simulink library "ITKLib"  (R2022b)
settings: Solver=FixedStepDiscrete  StartTime=0.0  StopTime=10.0  FixedStep=0.01  RelTol=1e-3  EnableMultiTasking=on
values from neighbouring files (symbols this model uses):
  Glb_WhlRollgRd_SC = single(0.36)    [init_Global.m]
undefined symbols (not defined in the file or in its folder): docblock, SlDemoSign, SlDemoSign_Positive_SC, TaskTime_100ms_SC, TaskTime_10ms_SC, VehRefSpd_vMaxRefSpd_C
libraries: simulink x51, $bdroot x45, ITKLib_V14 x1
(part 10 of 10)

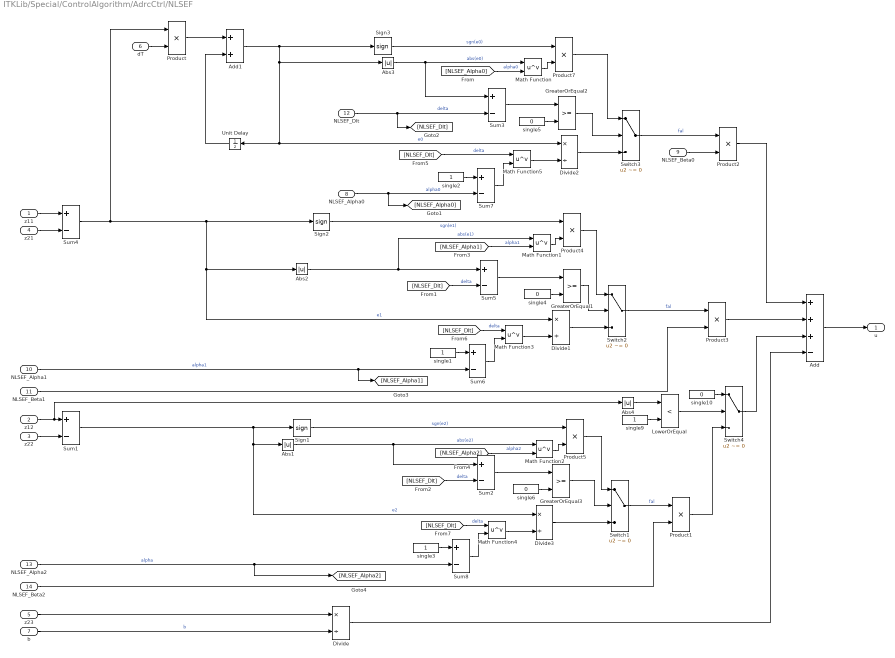
== system ITKLib/Special/ControlAlgorithm/AdrcCtrl/NLSEF ==
  z11 : Inport
  z12 : Inport  Port=2
  z22 : Inport  Port=3
  z21 : Inport  Port=4
  z23 : Inport  Port=5
  dT : Inport  Port=6
  b : Inport  Port=7
  NLSEF_Alpha0 : Inport  Port=8
  NLSEF_Beta0 : Inport  Port=9
  NLSEF_Alpha1 : Inport  Port=10
  NLSEF_Beta1 : Inport  Port=11
  NLSEF_Dlt : Inport  Port=12
  NLSEF_Alpha2 : Inport  Port=13
  NLSEF_Beta2 : Inport  Port=14
  Abs{1..4} (4 alike) : Abs  SaturateOnIntegerOverflow=off
  Add : Sum  Inputs=+++-
  Add1 : Sum
  Divide{,1..3} (4 alike) : Product  Inputs=*/  InputSameDT=on  SaturateOnIntegerOverflow=on
  GreaterOrEqual1 : RelationalOperator  OutDataTypeStr=boolean
  GreaterOrEqual2 : RelationalOperator  OutDataTypeStr=boolean
  GreaterOrEqual3 : RelationalOperator  OutDataTypeStr=boolean
  LowerOrEqual : RelationalOperator  Operator=<  OutDataTypeStr=boolean
  Math Function{,1..5} (6 alike) : Math  Operator=pow
  Product : Product  InputSameDT=on  SaturateOnIntegerOverflow=on
  Product1 : Product  RndMeth=Zero
  Product2 : Product  RndMeth=Zero
  Product3 : Product  RndMeth=Zero
  Product4 : Product
  Product5 : Product
  Product7 : Product
  Sign1 : Signum
  Sign2 : Signum
  Sign3 : Signum
  Sum{1..8} (8 alike) : Sum  Inputs=+-  SaturateOnIntegerOverflow=on
  Switch{1..4} (4 alike) : Switch  Criteria=u2 ~= 0  SaturateOnIntegerOverflow=off  InputSameDT=off
      Switch4 settings: AttributesFormatString=Criteria : %<Criteria>
  Unit Delay : UnitDelay  SampleTime=-1  HasFrameUpgradeWarning=on
  single{1..3,9} (4 alike) : Constant  OutDataTypeStr=single  SampleTime=-1
      settings: AttributesFormatString=%<OutDataTypeStr>
  single{4..6,10} (4 alike) : Constant  Value=0  OutDataTypeStr=single  SampleTime=-1
      settings: AttributesFormatString=%<OutDataTypeStr>
  u : Outport  VectorParamsAs1DForOutWhenUnconnected=off
  wires:
  Switch2/1 -> Product3/1  "fal"
  NLSEF_Alpha1/1 -> [NLSEF_Alpha1], Sum6/2  "alpha1"
  Product4/1 -> Switch2/1
  Abs2/1 -> Math Function1/1, Sum5/1  "abs(e1)"
  Divide1/1 -> Switch2/3
  Sum5/1 -> GreaterOrEqual1/1
  z11/1 -> Sum4/1
  [NLSEF_Dlt] -> Sum5/2  "delta"
  Sum4/1 -> Product/1, Sign2/1, Divide1/1, Abs2/1  "e1"
  Sign2/1 -> Product4/1  "sgn(e1)"
  NLSEF_Beta1/1 -> Product3/2
  z21/1 -> Sum4/2
  z22/1 -> Sum1/2
  NLSEF_Beta2/1 -> Product1/2
  Sign1/1 -> Product5/1  "sgn(e2)"
  Sum1/1 -> Sign1/1, Divide3/1, Abs1/1  "e2"
  [NLSEF_Dlt] -> Sum2/2  "delta"
  Divide3/1 -> Switch1/3
  Abs1/1 -> Math Function2/1, Sum2/1  "abs(e2)"
  NLSEF_Alpha2/1 -> [NLSEF_Alpha2], Sum8/2  "alpha"
  Sum2/1 -> GreaterOrEqual3/1
  Switch1/1 -> Product1/1  "fal"
  z12/1 -> Abs4/1, Sum1/1
  Product1/1 -> Switch4/3
  Product3/1 -> Add/2
  Product2/1 -> Add/1
  z23/1 -> Divide/1
  Divide/1 -> Add/4
  Add/1 -> u/1
  NLSEF_Dlt/1 -> Sum3/2, [NLSEF_Dlt]  "delta"
  Sign3/1 -> Product7/1  "sgn(e0)"
  NLSEF_Beta0/1 -> Product2/2
  Product7/1 -> Switch3/1
  Add1/1 -> Unit Delay/1, Divide2/1, Abs3/1, Sign3/1  "e0"
  Abs3/1 -> Math Function/1, Sum3/1  "abs(e0)"
  Sum3/1 -> GreaterOrEqual2/1
  Divide2/1 -> Switch3/3
  NLSEF_Alpha0/1 -> [NLSEF_Alpha0], Sum7/2  "alpha0"
  Switch3/1 -> Product2/1  "fal"
  [NLSEF_Alpha0] -> Math Function/2  "alpha0"
  [NLSEF_Alpha1] -> Math Function1/2  "alpha1"
  [NLSEF_Alpha2] -> Math Function2/2  "alpha2"
  b/1 -> Divide/2  "b"
  Unit Delay/1 -> Add1/2
  Product/1 -> Add1/1
  dT/1 -> Product/2
  Math Function/1 -> Product7/2
  Math Function1/1 -> Product4/2
  Math Function2/1 -> Product5/2
  Product5/1 -> Switch1/1
  single2/1 -> Sum7/1
  Math Function5/1 -> Divide2/2
  Sum7/1 -> Math Function5/2
  [NLSEF_Dlt] -> Math Function5/1  "delta"
  Sum6/1 -> Math Function3/2
  Math Function3/1 -> Divide1/2
  single1/1 -> Sum6/1
  [NLSEF_Dlt] -> Math Function3/1  "delta"
  [NLSEF_Dlt] -> Math Function4/1  "delta"
  single3/1 -> Sum8/1
  Math Function4/1 -> Divide3/2
  Sum8/1 -> Math Function4/2
  single5/1 -> GreaterOrEqual2/2
  GreaterOrEqual2/1 -> Switch3/2
  single4/1 -> GreaterOrEqual1/2
  GreaterOrEqual1/1 -> Switch2/2
  single6/1 -> GreaterOrEqual3/2
  GreaterOrEqual3/1 -> Switch1/2
  single10/1 -> Switch4/1
  LowerOrEqual/1 -> Switch4/2
  single9/1 -> LowerOrEqual/2
  Abs4/1 -> LowerOrEqual/1
  Switch4/1 -> Add/3

== system ITKLib/Special/ControlAlgorithm/AdrcCtrl/TD ==
  yd : Inport
  r : Inport  Port=2
  h : Inport  Port=3
  Ts : Inport  Port=4
  Abs : Abs  SaturateOnIntegerOverflow=off
  Abs1 : Abs  SaturateOnIntegerOverflow=off
  Add{,1..3} (4 alike) : Sum
  Divide : Product  Inputs=*/
  Divide1 : Product  Inputs=**/
  Divide2 : Product  Inputs=*/
  Gain : Gain  Gain=-1
  Gain1 : Gain  Gain=-1
  GreaterOrEqual1 : RelationalOperator  OutDataTypeStr=boolean
  GreaterOrEqual2 : RelationalOperator  OutDataTypeStr=boolean
  Product{,1..6,8} (8 alike) : Product  RndMeth=Zero
  Product7 : Product  Inputs=3  RndMeth=Zero
  Sign : Signum
  Sign1 : Signum
  Sqrt : $bdroot/BasicOperators/Sqrt
  Sum1 : Sum  Inputs=+-+  SaturateOnIntegerOverflow=on
  Sum2 : Sum  Inputs=+-  SaturateOnIntegerOverflow=on
  Sum3 : Sum  Inputs=+-  SaturateOnIntegerOverflow=on
  Sum4 : Sum  Inputs=+-  SaturateOnIntegerOverflow=on
  Switch : Switch  Criteria=u2 ~= 0  SaturateOnIntegerOverflow=off  InputSameDT=off
  Switch1 : Switch  Criteria=u2 ~= 0  SaturateOnIntegerOverflow=off  InputSameDT=off
  Unit Delay : UnitDelay  SampleTime=-1  HasFrameUpgradeWarning=on
  Unit Delay1 : UnitDelay  SampleTime=-1  HasFrameUpgradeWarning=on
  single : Constant  Value=2  OutDataTypeStr=single  SampleTime=-1
      settings: AttributesFormatString=%<OutDataTypeStr>
  single1 : Constant  Value=8  OutDataTypeStr=single  SampleTime=-1
      settings: AttributesFormatString=%<OutDataTypeStr>
  single2 : Constant  Value=0  OutDataTypeStr=single  SampleTime=-1
      settings: AttributesFormatString=%<OutDataTypeStr>
  single5 : Constant  Value=0  OutDataTypeStr=single  SampleTime=-1
      settings: AttributesFormatString=%<OutDataTypeStr>
  z11 : Outport  VectorParamsAs1DForOutWhenUnconnected=off
  z12 : Outport  Port=2  VectorParamsAs1DForOutWhenUnconnected=off
  wires:
  Product/1 -> Sum4/2, Product8/2, Product8/1, Divide1/3, Sum3/2, Product1/1  "d"
  r/1 -> [r], Product/1  "r"
  Switch1/1 -> Product4/1  "fhan"
  Add/1 -> Unit Delay/1  "y2(k+1)"
  h/1 -> Product/2, [h], Product3/2  "h"
  Abs/1 -> Product7/2, [y0abs]  "abs(y0)"
  Sum2/1 -> GreaterOrEqual2/1
  Sum3/1 -> GreaterOrEqual1/1
  Divide1/1 -> Gain1/1
  Product2/1 -> Gain/1
  Gain/1 -> Switch1/1
  yd/1 -> Sum1/2
  Sign1/1 -> Product2/1  "sgn(a)"
  Divide/1 -> Switch/3
  Sum1/1 -> [y0], Abs/1  "y0"
  Add2/1 -> Divide1/2, Abs1/1, Sign1/1  "a"
  Abs1/1 -> Sum3/1  "abs(a)"
  Sign/1 -> Product6/2  "sgn(y0)"
  Product1/1 -> Sum2/2  "d0"
  Sqrt/1 -> Sum4/1  "a0"
  Gain1/1 -> Switch1/3
  Product4/1 -> Add/1
  Unit Delay/1 -> Add/2, z12/1, [y2k]  "y2(k)"
  [y2k] -> Product5/1
  Product5/1 -> Add1/1
  Add1/1 -> Unit Delay1/1  "y1(k+1)"
  Unit Delay1/1 -> Add1/2, Sum1/1, z11/1  "y1(k)"
  [y2k] -> Product3/1
  Product3/1 -> Sum1/3
  Divide2/1 -> Switch/1
  Switch/1 -> Add2/2
  [y2k] -> Add2/1
  [y0abs] -> Sum2/1
  [y0] -> Sign/1
  [y0] -> Divide/1
  [r] -> Product2/2  "r"
  [r] -> Divide1/1  "r"
  [h] -> Divide/2, Product1/2  "h"
  Ts/1 -> [Ts], Product4/2
  [Ts] -> Product5/2
  Sum4/1 -> Product6/1
  Product6/1 -> Divide2/1
  single/1 -> Divide2/2
  single1/1 -> Product7/1
  Product7/1 -> Add3/1
  Product8/1 -> Add3/2
  Add3/1 -> Sqrt/1
  [r] -> Product7/3  "r"
  single5/1 -> GreaterOrEqual2/2
  GreaterOrEqual2/1 -> Switch/2
  single2/1 -> GreaterOrEqual1/2
  GreaterOrEqual1/1 -> Switch1/2

== system ITKLib/Special/ControlAlgorithm/RCCritCurr/Safe_Divide ==
  In : Inport
  In1 : Inport  Port=2
  eps : Inport  Port=3
  AND : Logic  OutDataTypeStr=boolean
  Abs : Abs  SaturateOnIntegerOverflow=off  OutDataTypeStr=Inherit: Inherit via internal rule
  Divide : Product  Inputs=*/  InputSameDT=on  SaturateOnIntegerOverflow=on
  GreaterOrEqual : RelationalOperator  OutDataTypeStr=boolean
  GreaterOrEqual1 : RelationalOperator  OutDataTypeStr=boolean
  LowerOrEqual : RelationalOperator  Operator=<=  OutDataTypeStr=boolean
  Opposite : Subsystem  RTWFcnName=Minus  RTWFileName=MCC_Mdl_Lib  mask(Opposite){}
      mask help:
      | output = - input;
      | Simulink Custom Model Library, created by MCC.
      settings: RTWFcnNameOpts=User specified  RTWFileNameOpts=User specified
      mask Display:
      | color('blue')
      | fprintf('-ln  ')
      | color('green');
      | % text(1,0,'SEN','horizontalAlignment','right','verticalAlignment','bottom');
  Opposite1 : Subsystem  RTWFcnName=Minus  RTWFileName=MCC_Mdl_Lib  mask(Opposite){}
      mask help:
      | output = - input;
      | Simulink Custom Model Library, created by MCC.
      settings: RTWFcnNameOpts=User specified  RTWFileNameOpts=User specified
      mask Display:
      | color('blue')
      | fprintf('-ln  ')
      | color('green');
      | % text(1,0,'SEN','horizontalAlignment','right','verticalAlignment','bottom');
  Switch : Switch  Criteria=u2 ~= 0  SaturateOnIntegerOverflow=off  InputSameDT=off
      settings: AttributesFormatString=Criteria : %<Criteria>
  Switch1 : Switch  Criteria=u2 ~= 0  SaturateOnIntegerOverflow=off  InputSameDT=off
      settings: AttributesFormatString=Criteria : %<Criteria>
  single : Constant  Value=0  OutDataTypeStr=single
      settings: AttributesFormatString=%<OutDataTypeStr>
  Out : Outport
  wires:
  Divide/1 -> Out/1
  In/1 -> Divide/1
  Switch/1 -> Divide/2
  AND/1 -> Switch/2
  In1/1 -> GreaterOrEqual/1, Switch/3, LowerOrEqual/1, GreaterOrEqual1/1
  single/1 -> GreaterOrEqual1/2
  eps/1 -> Abs/1
  Abs/1 -> [epsAbs], LowerOrEqual/2
  LowerOrEqual/1 -> AND/1
  GreaterOrEqual/1 -> AND/2
  Opposite/1(" Out ") -> GreaterOrEqual/2
  [epsAbs] -> Opposite/1(In)
  GreaterOrEqual1/1 -> Switch1/2
  [epsAbs] -> Opposite1/1(In)
  Opposite1/1(" Out ") -> Switch1/3
  [epsAbs] -> Switch1/1
  Switch1/1 -> Switch/1

== system ITKLib/Special/ControlAlgorithm/RCCritCurr/Safe_Divide/Opposite ==
  In : Inport
  Product2 : Product  InputSameDT=on  SaturateOnIntegerOverflow=on
  single : Constant  Value=-1  OutDataTypeStr=single
      settings: AttributesFormatString=%<OutDataTypeStr>
  " Out " : Outport
  wires:
  single/1 -> Product2/2
  Product2/1 -> " Out "/1
  In/1 -> Product2/1

== system ITKLib/Special/ControlAlgorithm/RCCritCurr/Safe_Divide/Opposite1 ==
  In : Inport
  Product2 : Product  InputSameDT=on  SaturateOnIntegerOverflow=on
  single : Constant  Value=-1  OutDataTypeStr=single
      settings: AttributesFormatString=%<OutDataTypeStr>
  " Out " : Outport
  wires:
  single/1 -> Product2/2
  Product2/1 -> " Out "/1
  In/1 -> Product2/1

== stateflow chart ITKLib/BasicOperators/Chart ==
  settings: updateMethod=DISCRETE

== matlab function ITKLib/Diagnosis/Crc8Gen ==
  data: MsgData input; CRCVal output; ChkLen input; Poly input; InitVal input; XORVal input
%% CRC8校验算法：生成CRC8 Checksum的Value数值
% Input signals：
%               MsgData:包含8个byte的完整的一个ID的报文数据包
%               ChkLen:进行校验的ID数据长度对应的数值，通常为固定值7个byte对应01111111对应的uint8为127
%               Poly:多项式Polynomial值，此处可以设置为16进制对应的十进制uint8数值
%               InitVal:初始值，此处可以设置为16进制对应的十进制uint8数值
%               XORVal:结果异或值XOROUT，此处可以设置为16进制对应的十进制uint8数值

%% 主函数
function CRCVal = Crc8Gen(MsgData,ChkLen,Poly,InitVal,XORVal)
crc = InitVal;
for i = 1:length(MsgData)
    if bitget(ChkLen,i) == 1
        crc = bitxor(crc,MsgData(i));
        for j = 0:7
            if bitand(crc,0x80) ~= 0
                crc = bitxor(bitshift(crc,1),Poly);
            else
                crc = bitshift(crc,1); 
            end
        end
    end
end
CRCVal = bitxor(crc,XORVal);
end

== matlab function ITKLib/BitOperation/GetBitU16/MATLAB Function ==
  data: u input; y output; mode input; N input
function y = fcn(u, mode, N)
%#codegen

switch mode
    case 1 % 逻辑左移 Shift Left Logical
        y = bitsll(cast_to_fi(u), N);
    case 2  % 逻辑右移 Shift Right Logical
        y = bitsrl(cast_to_fi(u), N);
%     case 3 % 算数右移 Shift Right Arithmetic
%         y = bitsra(cast_to_fi(u), N);
    otherwise
        y = cast_to_fi(u);
end

== matlab function ITKLib/BitOperation/GetBitU16/MATLAB Function1 ==
  data: u input; y output; mode input; N input
function y = fcn(u, mode, N)
%#codegen

switch mode
    case 1 % 逻辑左移 Shift Left Logical
        y = bitsll(cast_to_fi(u), N);
    case 2  % 逻辑右移 Shift Right Logical
        y = bitsrl(cast_to_fi(u), N);
%     case 3 % 算数右移 Shift Right Arithmetic
%         y = bitsra(cast_to_fi(u), N);
    otherwise
        y = cast_to_fi(u);
end

== matlab function ITKLib/BitOperation/GetBitU8/MATLAB Function ==
  data: u input; y output; mode input; N input
function y = fcn(u, mode, N)
%#codegen

switch mode
    case 1 % 逻辑左移 Shift Left Logical，尽量选择逻辑左移或右移
        y = bitsll(cast_to_fi(u), N);
    case 2  % 逻辑右移 Shift Right Logical
        y = bitsrl(cast_to_fi(u), N);
%     case 3 % 算数右移 Shift Right Arithmetic
%         y = bitsra(cast_to_fi(u), N);
    otherwise
        y = cast_to_fi(u);
end

== matlab function ITKLib/BitOperation/GetBitU8/MATLAB Function1 ==
  data: u input; y output; mode input; N input
function y = fcn(u, mode, N)
%#codegen

switch mode
    case 1 % 逻辑左移 Shift Left Logical
        y = bitsll(cast_to_fi(u), N);
    case 2  % 逻辑右移 Shift Right Logical
        y = bitsrl(cast_to_fi(u), N);
%     case 3 % 算数右移 Shift Right Arithmetic
%         y = bitsra(cast_to_fi(u), N);
    otherwise
        y = cast_to_fi(u);
end

== matlab function ITKLib/BitOperation/GetBitU32/MATLAB Function ==
  data: u input; y output; mode input; N input
function y = fcn(u, mode, N)
%#codegen

switch mode
    case 1 % 逻辑左移 Shift Left Logical
        y = bitsll(cast_to_fi(u), N);
    case 2  % 逻辑右移 Shift Right Logical
        y = bitsrl(cast_to_fi(u), N);
%     case 3 % 算数右移 Shift Right Arithmetic
%         y = bitsra(cast_to_fi(u), N);
    otherwise
        y = cast_to_fi(u);
end

== matlab function ITKLib/BitOperation/GetBitU32/MATLAB Function1 ==
  data: u input; y output; mode input; N input
function y = fcn(u, mode, N)
%#codegen

switch mode
    case 1 % 逻辑左移 Shift Left Logical
        y = bitsll(cast_to_fi(u), N);
    case 2  % 逻辑右移 Shift Right Logical
        y = bitsrl(cast_to_fi(u), N);
%     case 3 % 算数右移 Shift Right Arithmetic
%         y = bitsra(cast_to_fi(u), N);
    otherwise
        y = cast_to_fi(u);
end

== stateflow chart ITKLib/Filter/MovgMinMaxAvrg ==
  (default) -> (junction 40) : {
      | /* Buffer new running average result */
      | InBufAry[idx] = In;
      | /* Increment persistent buffer pointer */
      | idx++;
      | /* Initialise FOR loop */
      | idx_loop = uint16(0);
      | Min = single(999999999999999999);
      | Max = single(-999999999999999999);
      | Avrg = single(0);
      | Sum = single(0);
      | }
  (junction 40) -> (junction 54) [order 1] : [idx_loop < DataNr]
  (junction 54) -> (junction 53) [order 1] : [InBufAry[idx_loop] > Max]
  (junction 102) -> (junction 40) : {idx_loop++;}
  (junction 40) -> (junction 7) [order 2] : {
      | /* Average the totals for input */
      | Avrg = Sum / DataNr;
      | }
  (junction 54) -> (junction 103) [order 2]
  (junction 53) -> (junction 52) : {
      | Max = InBufAry[idx_loop];
      | }
  (junction 103) -> (junction 105) [order 1] : [InBufAry[idx_loop] < Min]
  (junction 103) -> (junction 55) [order 2]
  (junction 105) -> (junction 107) : {
      | Min = InBufAry[idx_loop];
      | }
  (junction 107) -> (junction 55)
  (junction 52) -> (junction 107)
  (junction 55) -> (junction 102) : {
      | Sum = Sum+InBufAry[idx_loop];
      | }
  (junction 7) -> (junction 10) [order 1] : /* Ring buffer pointer has reached end of ring */
      | [idx == DataNr]
  (junction 7) -> (junction 9) [order 2]
  (junction 10) -> (junction 11) : /* Reset pointer to start of buffer */
      | {idx = uint16(0);}
  (junction 11) -> (junction 9)
  data: In input single; InBufAry local single size=[1 DataNr]; idx local uint16 size=1 =0; DataNr input uint16; idx_loop local uint16 size=1 =0; Sum local single; Min output single; Max output single; Avrg output single; data local single

== stateflow chart ITKLib/TimeCounter/trig_TaskTime_A ==
  settings: updateMethod=DISCRETE
  (default) -> (junction 52) : {cnt = cnt + 1;}
  (junction 52) -> (junction 54) [order 1] : [cnt %% 2 == 0]
  (junction 52) -> (junction 58) [order 2]
  (junction 54) -> (junction 56) : {
      |   trig_TaskTime_20ms;
      | }
  (junction 56) -> (junction 58)
  (junction 58) -> (junction 83)
  (junction 83) -> (junction 81) [order 1] : [cnt %% 5 == 0]
  (junction 83) -> (junction 87) [order 2]
  (junction 81) -> (junction 82) : {
      |   trig_TaskTime_50ms;
      | }
  (junction 82) -> (junction 87)
  (junction 87) -> (junction 96)
  (junction 96) -> (junction 90) [order 1] : [cnt %% 10 == 0]
  (junction 96) -> (junction 95) [order 2]
  (junction 90) -> (junction 93) : {
      |   trig_TaskTime_100ms;
      | }
  (junction 93) -> (junction 95)
  (junction 95) -> (junction 111)
  (junction 111) -> (junction 114) [order 1] : [cnt %% 20 == 0]
  (junction 111) -> (junction 110) [order 2]
  (junction 114) -> (junction 108) : {
      |   trig_TaskTime_200ms;
      | }
  (junction 108) -> (junction 110)
  (junction 110) -> (junction 118)
  (junction 118) -> (junction 120) [order 1] : [cnt %% 50 == 0]
  (junction 118) -> (junction 117) [order 2]
  (junction 120) -> (junction 124) : {
      |   trig_TaskTime_500ms;
      | }
  (junction 124) -> (junction 117)
  (junction 117) -> (junction 128)
  (junction 128) -> (junction 132) [order 1] : [cnt %% 100 == 0]
  (junction 128) -> (junction 131) [order 2]
  (junction 132) -> (junction 126) : {
      |   trig_TaskTime_1000ms;
      |   cnt = 0;
      | }
  (junction 126) -> (junction 131)
  (junction 131) -> (junction 20)
  data: cnt local uint16
  events: trig_TaskTime_20ms output FUNCTION_CALL_EVENT; trig_TaskTime_50ms output FUNCTION_CALL_EVENT; trig_TaskTime_100ms output FUNCTION_CALL_EVENT; trig_TaskTime_200ms output FUNCTION_CALL_EVENT; trig_TaskTime_500ms output FUNCTION_CALL_EVENT; trig_TaskTime_1000ms output FUNCTION_CALL_EVENT

== stateflow chart ITKLib/TimeCounter/trig_TaskTime_B ==
  settings: updateMethod=DISCRETE
  (default) -> (junction 52) : {cnt = cnt + 1;}
  (junction 52) -> (junction 54) [order 1] : [cnt %% 3 == 0]
  (junction 52) -> (junction 58) [order 2]
  (junction 54) -> (junction 56) : {
      |   trig_TaskTime_30ms;
      | }
  (junction 56) -> (junction 58)
  (junction 58) -> (junction 83)
  (junction 83) -> (junction 81) [order 1] : [cnt %% 15 == 0]
  (junction 83) -> (junction 87) [order 2]
  (junction 81) -> (junction 82) : {
      |   trig_TaskTime_150ms;
      | }
  (junction 82) -> (junction 87)
  (junction 87) -> (junction 96)
  (junction 96) -> (junction 90) [order 1] : [cnt %% 30 == 0]
  (junction 96) -> (junction 95) [order 2]
  (junction 90) -> (junction 93) : {
      |   trig_TaskTime_300ms;
      |   cnt = 0;
      | }
  (junction 93) -> (junction 95)
  (junction 95) -> (junction 20)
  data: cnt local uint16
  events: trig_TaskTime_30ms output FUNCTION_CALL_EVENT; trig_TaskTime_150ms output FUNCTION_CALL_EVENT; trig_TaskTime_300ms output FUNCTION_CALL_EVENT

== stateflow chart ITKLib/Diagnosis/FltCollctn/FltStAry ==
  settings: updateMethod=DISCRETE
  (default) -> (junction 233)
  (junction 233) -> (junction 257) : {BatProt_stFltAry[FltNr-1] = (BatProt_stFltAry[FltNr-1] & 0xFD);}
  (junction 257) -> (junction 265)
  (junction 265) -> (junction 244) : {BatProt_stFltAry[FltNr-1] = (BatProt_stFltAry[FltNr-1] & 0xF7);}
  (junction 244) -> (junction 250)
  (junction 250) -> (junction 266) [order 1] : [FltFlg==1]{BatProt_stFltAry[FltNr-1] = (BatProt_stFltAry[FltNr-1] | 0x10);}
  (junction 250) -> (junction 252) [order 2] : {BatProt_stFltAry[FltNr-1] = (BatProt_stFltAry[FltNr-1] & 0xEF);}
  (junction 266) -> (junction 246)
  (junction 246) -> (junction 252)
  (junction 252) -> (junction 239)
  (junction 239) -> (junction 258) : {BatProt_stFltAry[FltNr-1] = (BatProt_stFltAry[FltNr-1] & 0xFB);}
  data: FltNr input uint8; BatProt_stFltAry data_store_memory size=4; FltFlg input boolean

== stateflow chart ITKLib/Diagnosis/FltCollctn/FltStCodAry ==
  settings: updateMethod=DISCRETE
  (default) -> (junction 13)
  (junction 13) -> (junction 15) [order 1] : [FltFlg]
  (junction 15) -> (junction 19) [order 1] : [BitPos==0]{BatProt_stFltCodAry[AryIdx]=(BatProt_stFltCodAry[AryIdx] | 0x1);}
  (junction 13) -> (junction 136) [order 2]
  (junction 15) -> (junction 22) [order 2]
  (junction 19) -> (junction 21)
  (junction 22) -> (junction 21) [order 1] : [BitPos==1]{BatProt_stFltCodAry[AryIdx]=(BatProt_stFltCodAry[AryIdx] | 0x2);}
  (junction 22) -> (junction 30) [order 2]
  (junction 21) -> (junction 32)
  (junction 136) -> (junction 166) [order 1] : [BitPos==0]{BatProt_stFltCodAry[AryIdx]=(BatProt_stFltCodAry[AryIdx] & 0xFFFE);}
  (junction 30) -> (junction 32) [order 1] : [BitPos==2]{BatProt_stFltCodAry[AryIdx]=(BatProt_stFltCodAry[AryIdx] | 0x4);}
  (junction 136) -> (junction 177) [order 2]
  (junction 166) -> (junction 169)
  (junction 30) -> (junction 39) [order 2]
  (junction 32) -> (junction 36)
  (junction 39) -> (junction 36) [order 1] : [BitPos==3]{BatProt_stFltCodAry[AryIdx]=(BatProt_stFltCodAry[AryIdx] | 0x8);}
  (junction 177) -> (junction 169) [order 1] : [BitPos==1]{BatProt_stFltCodAry[AryIdx]=(BatProt_stFltCodAry[AryIdx] & 0xFFFD);}
  (junction 39) -> (junction 42) [order 2]
  (junction 36) -> (junction 50)
  (junction 177) -> (junction 179) [order 2]
  (junction 169) -> (junction 138)
  (junction 179) -> (junction 138) [order 1] : [BitPos==2]{BatProt_stFltCodAry[AryIdx]=(BatProt_stFltCodAry[AryIdx] & 0xFFFB);}
  (junction 42) -> (junction 50) [order 1] : [BitPos==4]{BatProt_stFltCodAry[AryIdx]=(BatProt_stFltCodAry[AryIdx] | 0x10);}
  (junction 179) -> (junction 122) [order 2]
  (junction 138) -> (junction 163)
  (junction 42) -> (junction 44) [order 2]
  (junction 50) -> (junction 46)
  (junction 122) -> (junction 163) [order 1] : [BitPos==3]{BatProt_stFltCodAry[AryIdx]=(BatProt_stFltCodAry[AryIdx] & 0xFFF7);}
  (junction 44) -> (junction 46) [order 1] : [BitPos==5]{BatProt_stFltCodAry[AryIdx]=(BatProt_stFltCodAry[AryIdx] | 0x20);}
  (junction 122) -> (junction 130) [order 2]
  (junction 163) -> (junction 109)
  (junction 44) -> (junction 45) [order 2]
  (junction 46) -> (junction 49)
  (junction 45) -> (junction 49) [order 1] : [BitPos==6]{BatProt_stFltCodAry[AryIdx]=(BatProt_stFltCodAry[AryIdx] | 0x40);}
  (junction 130) -> (junction 109) [order 1] : [BitPos==4]{BatProt_stFltCodAry[AryIdx]=(BatProt_stFltCodAry[AryIdx] & 0xFFEF);}
  (junction 45) -> (junction 64) [order 2]
  (junction 49) -> (junction 81)
  (junction 130) -> (junction 111) [order 2]
  (junction 109) -> (junction 175)
  (junction 64) -> (junction 81) [order 1] : [BitPos==7]{BatProt_stFltCodAry[AryIdx]=(BatProt_stFltCodAry[AryIdx] | 0x80);}
  (junction 64) -> (junction 67) [order 2]
  (junction 81) -> (junction 75)
  (junction 111) -> (junction 175) [order 1] : [BitPos==5]{BatProt_stFltCodAry[AryIdx]=(BatProt_stFltCodAry[AryIdx] & 0xFFDF);}
  (junction 111) -> (junction 121) [order 2]
  (junction 175) -> (junction 105)
  (junction 67) -> (junction 75) [order 1] : [BitPos==8]{BatProt_stFltCodAry[AryIdx]=(BatProt_stFltCodAry[AryIdx] | 0x100);}
  (junction 67) -> (junction 69) [order 2]
  (junction 75) -> (junction 79)
  (junction 121) -> (junction 105) [order 1] : [BitPos==6]{BatProt_stFltCodAry[AryIdx]=(BatProt_stFltCodAry[AryIdx] & 0xFFBF);}
  (junction 121) -> (junction 104) [order 2]
  (junction 105) -> (junction 143)
  (junction 69) -> (junction 79) [order 1] : [BitPos==9]{BatProt_stFltCodAry[AryIdx]=(BatProt_stFltCodAry[AryIdx] | 0x200);}
  (junction 104) -> (junction 143) [order 1] : [BitPos==7]{BatProt_stFltCodAry[AryIdx]=(BatProt_stFltCodAry[AryIdx] & 0xFF7F);}
  (junction 69) -> (junction 71) [order 2]
  (junction 79) -> (junction 57)
  (junction 104) -> (junction 171) [order 2]
  (junction 143) -> (junction 110)
  (junction 71) -> (junction 57) [order 1] : [BitPos==10]{BatProt_stFltCodAry[AryIdx]=(BatProt_stFltCodAry[AryIdx] | 0x400);}
  (junction 171) -> (junction 110) [order 1] : [BitPos==8]{BatProt_stFltCodAry[AryIdx]=(BatProt_stFltCodAry[AryIdx] & 0xFEFF);}
  (junction 71) -> (junction 59) [order 2]
  (junction 57) -> (junction 63)
  (junction 171) -> (junction 149) [order 2]
  (junction 110) -> (junction 145)
  (junction 59) -> (junction 63) [order 1] : [BitPos==11]{BatProt_stFltCodAry[AryIdx]=(BatProt_stFltCodAry[AryIdx] | 0x800);}
  (junction 149) -> (junction 145) [order 1] : [BitPos==9]{BatProt_stFltCodAry[AryIdx]=(BatProt_stFltCodAry[AryIdx] & 0xFDFF);}
  (junction 59) -> (junction 68) [order 2]
  (junction 63) -> (junction 55)
  (junction 149) -> (junction 176) [order 2]
  (junction 145) -> (junction 131)
  (junction 68) -> (junction 55) [order 1] : [BitPos==12]{BatProt_stFltCodAry[AryIdx]=(BatProt_stFltCodAry[AryIdx] | 0x1000);}
  (junction 176) -> (junction 131) [order 1] : [BitPos==10]{BatProt_stFltCodAry[AryIdx]=(BatProt_stFltCodAry[AryIdx] & 0xFBFF);}
  (junction 68) -> (junction 98) [order 2]
  (junction 55) -> (junction 95)
  (junction 176) -> (junction 142) [order 2]
  (junction 131) -> (junction 106)
  (junction 98) -> (junction 95) [order 1] : [BitPos==13]{BatProt_stFltCodAry[AryIdx]=(BatProt_stFltCodAry[AryIdx] | 0x2000);}
  (junction 142) -> (junction 106) [order 1] : [BitPos==11]{BatProt_stFltCodAry[AryIdx]=(BatProt_stFltCodAry[AryIdx] & 0xF7FF);}
  (junction 98) -> (junction 90) [order 2]
  (junction 95) -> (junction 89)
  (junction 142) -> (junction 103) [order 2]
  (junction 106) -> (junction 146)
  (junction 90) -> (junction 89) [order 1] : [BitPos==14]{BatProt_stFltCodAry[AryIdx]=(BatProt_stFltCodAry[AryIdx] | 0x4000);}
  (junction 103) -> (junction 146) [order 1] : [BitPos==12]{BatProt_stFltCodAry[AryIdx]=(BatProt_stFltCodAry[AryIdx] & 0xEFFF);}
  (junction 90) -> (junction 91) [order 2]
  (junction 89) -> (junction 97)
  (junction 103) -> (junction 118) [order 2]
  (junction 146) -> (junction 178)
  (junction 91) -> (junction 97) [order 1] : [BitPos==15]{BatProt_stFltCodAry[AryIdx]=(BatProt_stFltCodAry[AryIdx] | 0x8000);}
  (junction 118) -> (junction 178) [order 1] : [BitPos==13]{BatProt_stFltCodAry[AryIdx]=(BatProt_stFltCodAry[AryIdx] & 0xDFFF);}
  (junction 91) -> (junction 189) [order 2]
  (junction 97) -> (junction 186)
  (junction 118) -> (junction 173) [order 2]
  (junction 178) -> (junction 134)
  (junction 173) -> (junction 134) [order 1] : [BitPos==14]{BatProt_stFltCodAry[AryIdx]=(BatProt_stFltCodAry[AryIdx] & 0xBFFF);}
  (junction 173) -> (junction 174) [order 2]
  (junction 134) -> (junction 156)
  (junction 174) -> (junction 156) [order 1] : [BitPos==15]{BatProt_stFltCodAry[AryIdx]=(BatProt_stFltCodAry[AryIdx] & 0x7FFF);}
  (junction 174) -> (junction 181) [order 2]
  (junction 156) -> (junction 183)
  (junction 181) -> (junction 183)
  (junction 183) -> (junction 189)
  (junction 189) -> (junction 186)
  data: FltFlg input boolean; AryIdx input uint8; BitPos input uint8; BatProt_stFltCodAry data_store_memory size=4

== matlab function ITKLib/Diagnosis/Crc16Gen ==
  data: MsgData input; CRCVal output; Poly input; InitVal input; xor_value input
%% CRC16_CCITT_False 校验算法：生成CRC16 Checksum的Value数值
% Input signals：
%               MsgData:包含32个byte的完整的一个ID的报文数据包
%               Poly:多项式Polynomial值，此处可以设置为16进制对应的十进制uint16数值
%               InitVal:初始值，此处可以设置为16进制对应的十进制uint16数值
%               XORVal:结果异或值XOROUT，此处可以设置为16进制对应的十进制uint16数值

%% 主函数 
function CRCVal = Crc16Gen(MsgData,Poly,InitVal,xor_value)

    % CRC 计算
    CRCVal = InitVal;
    for i = 1:length(MsgData)
        byte = uint16(MsgData(i));
        CRCVal = bitxor(CRCVal, bitshift(byte, 8));  % 将当前字节左移8位后与CRC异或
        
        % 处理8位
        for j = 1:8
            if bitand(CRCVal, hex2dec('8000'))  % 检查最高位
                CRCVal = bitxor(bitshift(CRCVal, 1), Poly);
            else
                CRCVal = bitshift(CRCVal, 1);
            end
            CRCVal = bitand(CRCVal, hex2dec('FFFF'));  % 保持16位
        end
    end
    
    % 异或操作（根据参数，这里为 0x0000，可以省略）
    CRCVal = bitxor(CRCVal, xor_value);

end

== stateflow chart ITKLib/TimeCounter/InDly ==
  (default) -> (junction 114)
  (junction 114) -> (junction 118) [order 1] : [i<DlyCnt]
  (junction 118) -> (junction 115) [order 1] : [i == DlyCnt-uint16(1)]
  (junction 115) -> (junction 116) : {/*output:delayed result*/
      | InDlyAry[DlyCnt-1] = In;
      | }
  (junction 116) -> (junction 114) : {
      | i++;
      | }
  (junction 114) -> (junction 117) [order 2] : {/*output:delayed result*/
      | InDly = InDlyAry[0];
      | i = uint16(0);
      | }
  (junction 118) -> (junction 116) [order 2] : {/*output:delayed result*/
      | InDlyAry[i] = InDlyAry[i+1];
      | }
  (junction 117) -> (junction 120) [order 1] : [j < DlyCnt]
  (junction 121) -> (junction 117) : {
      | j++;
      | }
  (junction 117) -> (junction 127) [order 2]
  (junction 120) -> (junction 121) : {
      | InDly = In;
      | }
  data: In input single; InDlyAry local single size=[1 610]; i local uint16 size=1 =0; DlyCnt input uint16; j local uint16 size=1 =0; InDly output single

== matlab function ITKLib/Special/ControlAlgorithm/QrCalc ==
  data: In input; Out output
function Out  = QrCalc(In)
%UNTITLED 此处显示有关此函数的摘要
%   此处显示详细说明
Out  = qr(In);
end

== matlab function ITKLib/Special/ControlAlgorithm/SvdCalc ==
  data: In input; Out output
function Out  = SvdCalc(In)
%UNTITLED 此处显示有关此函数的摘要
%   此处显示详细说明
[Out,~,~] = svd(In);
end

== stateflow chart ITKLib/Diagnosis/FltLatchCollctn/FltStAry ==
  settings: updateMethod=DISCRETE
  (default) -> (junction 233)
  (junction 233) -> (junction 257) : {BatProt_stFltAry[FltNr-1] = (BatProt_stFltAry[FltNr-1] & 0xFD);}
  (junction 257) -> (junction 265)
  (junction 265) -> (junction 244) : {BatProt_stFltAry[FltNr-1] = (BatProt_stFltAry[FltNr-1] & 0xF7);}
  (junction 244) -> (junction 250)
  (junction 250) -> (junction 266) [order 1] : [FltFlg==1]{BatProt_stFltAry[FltNr-1] = (BatProt_stFltAry[FltNr-1] | 0x10);}
  (junction 250) -> (junction 252) [order 2] : {BatProt_stFltAry[FltNr-1] = (BatProt_stFltAry[FltNr-1] & 0xEF);}
  (junction 266) -> (junction 246)
  (junction 246) -> (junction 252)
  (junction 252) -> (junction 239)
  (junction 239) -> (junction 258) : {BatProt_stFltAry[FltNr-1] = (BatProt_stFltAry[FltNr-1] & 0xFB);}
  data: FltNr input uint8; BatProt_stFltAry data_store_memory size=4; FltFlg input boolean

== stateflow chart ITKLib/Diagnosis/FltLatchCollctn/FltStCodAry ==
  settings: updateMethod=DISCRETE
  (default) -> (junction 13)
  (junction 13) -> (junction 15) [order 1] : [FltFlg]
  (junction 15) -> (junction 19) [order 1] : [BitPos==0]{BatProt_stFltCodAry[AryIdx]=(BatProt_stFltCodAry[AryIdx] | 0x1);}
  (junction 13) -> (junction 136) [order 2]
  (junction 15) -> (junction 22) [order 2]
  (junction 19) -> (junction 21)
  (junction 22) -> (junction 21) [order 1] : [BitPos==1]{BatProt_stFltCodAry[AryIdx]=(BatProt_stFltCodAry[AryIdx] | 0x2);}
  (junction 22) -> (junction 30) [order 2]
  (junction 21) -> (junction 32)
  (junction 136) -> (junction 166) [order 1] : [BitPos==0]{BatProt_stFltCodAry[AryIdx]=(BatProt_stFltCodAry[AryIdx] & 0xFFFE);}
  (junction 30) -> (junction 32) [order 1] : [BitPos==2]{BatProt_stFltCodAry[AryIdx]=(BatProt_stFltCodAry[AryIdx] | 0x4);}
  (junction 136) -> (junction 177) [order 2]
  (junction 166) -> (junction 169)
  (junction 30) -> (junction 39) [order 2]
  (junction 32) -> (junction 36)
  (junction 39) -> (junction 36) [order 1] : [BitPos==3]{BatProt_stFltCodAry[AryIdx]=(BatProt_stFltCodAry[AryIdx] | 0x8);}
  (junction 177) -> (junction 169) [order 1] : [BitPos==1]{BatProt_stFltCodAry[AryIdx]=(BatProt_stFltCodAry[AryIdx] & 0xFFFD);}
  (junction 39) -> (junction 42) [order 2]
  (junction 36) -> (junction 50)
  (junction 177) -> (junction 179) [order 2]
  (junction 169) -> (junction 138)
  (junction 179) -> (junction 138) [order 1] : [BitPos==2]{BatProt_stFltCodAry[AryIdx]=(BatProt_stFltCodAry[AryIdx] & 0xFFFB);}
  (junction 42) -> (junction 50) [order 1] : [BitPos==4]{BatProt_stFltCodAry[AryIdx]=(BatProt_stFltCodAry[AryIdx] | 0x10);}
  (junction 179) -> (junction 122) [order 2]
  (junction 138) -> (junction 163)
  (junction 42) -> (junction 44) [order 2]
  (junction 50) -> (junction 46)
  (junction 122) -> (junction 163) [order 1] : [BitPos==3]{BatProt_stFltCodAry[AryIdx]=(BatProt_stFltCodAry[AryIdx] & 0xFFF7);}
  (junction 44) -> (junction 46) [order 1] : [BitPos==5]{BatProt_stFltCodAry[AryIdx]=(BatProt_stFltCodAry[AryIdx] | 0x20);}
  (junction 122) -> (junction 130) [order 2]
  (junction 163) -> (junction 109)
  (junction 44) -> (junction 45) [order 2]
  (junction 46) -> (junction 49)
  (junction 45) -> (junction 49) [order 1] : [BitPos==6]{BatProt_stFltCodAry[AryIdx]=(BatProt_stFltCodAry[AryIdx] | 0x40);}
  (junction 130) -> (junction 109) [order 1] : [BitPos==4]{BatProt_stFltCodAry[AryIdx]=(BatProt_stFltCodAry[AryIdx] & 0xFFEF);}
  (junction 45) -> (junction 64) [order 2]
  (junction 49) -> (junction 81)
  (junction 130) -> (junction 111) [order 2]
  (junction 109) -> (junction 175)
  (junction 64) -> (junction 81) [order 1] : [BitPos==7]{BatProt_stFltCodAry[AryIdx]=(BatProt_stFltCodAry[AryIdx] | 0x80);}
  (junction 64) -> (junction 67) [order 2]
  (junction 81) -> (junction 75)
  (junction 111) -> (junction 175) [order 1] : [BitPos==5]{BatProt_stFltCodAry[AryIdx]=(BatProt_stFltCodAry[AryIdx] & 0xFFDF);}
  (junction 111) -> (junction 121) [order 2]
  (junction 175) -> (junction 105)
  (junction 67) -> (junction 75) [order 1] : [BitPos==8]{BatProt_stFltCodAry[AryIdx]=(BatProt_stFltCodAry[AryIdx] | 0x100);}
  (junction 67) -> (junction 69) [order 2]
  (junction 75) -> (junction 79)
  (junction 121) -> (junction 105) [order 1] : [BitPos==6]{BatProt_stFltCodAry[AryIdx]=(BatProt_stFltCodAry[AryIdx] & 0xFFBF);}
  (junction 121) -> (junction 104) [order 2]
  (junction 105) -> (junction 143)
  (junction 69) -> (junction 79) [order 1] : [BitPos==9]{BatProt_stFltCodAry[AryIdx]=(BatProt_stFltCodAry[AryIdx] | 0x200);}
  (junction 104) -> (junction 143) [order 1] : [BitPos==7]{BatProt_stFltCodAry[AryIdx]=(BatProt_stFltCodAry[AryIdx] & 0xFF7F);}
  (junction 69) -> (junction 71) [order 2]
  (junction 79) -> (junction 57)
  (junction 104) -> (junction 171) [order 2]
  (junction 143) -> (junction 110)
  (junction 71) -> (junction 57) [order 1] : [BitPos==10]{BatProt_stFltCodAry[AryIdx]=(BatProt_stFltCodAry[AryIdx] | 0x400);}
  (junction 171) -> (junction 110) [order 1] : [BitPos==8]{BatProt_stFltCodAry[AryIdx]=(BatProt_stFltCodAry[AryIdx] & 0xFEFF);}
  (junction 71) -> (junction 59) [order 2]
  (junction 57) -> (junction 63)
  (junction 171) -> (junction 149) [order 2]
  (junction 110) -> (junction 145)
  (junction 59) -> (junction 63) [order 1] : [BitPos==11]{BatProt_stFltCodAry[AryIdx]=(BatProt_stFltCodAry[AryIdx] | 0x800);}
  (junction 149) -> (junction 145) [order 1] : [BitPos==9]{BatProt_stFltCodAry[AryIdx]=(BatProt_stFltCodAry[AryIdx] & 0xFDFF);}
  (junction 59) -> (junction 68) [order 2]
  (junction 63) -> (junction 55)
  (junction 149) -> (junction 176) [order 2]
  (junction 145) -> (junction 131)
  (junction 68) -> (junction 55) [order 1] : [BitPos==12]{BatProt_stFltCodAry[AryIdx]=(BatProt_stFltCodAry[AryIdx] | 0x1000);}
  (junction 176) -> (junction 131) [order 1] : [BitPos==10]{BatProt_stFltCodAry[AryIdx]=(BatProt_stFltCodAry[AryIdx] & 0xFBFF);}
  (junction 68) -> (junction 98) [order 2]
  (junction 55) -> (junction 95)
  (junction 176) -> (junction 142) [order 2]
  (junction 131) -> (junction 106)
  (junction 98) -> (junction 95) [order 1] : [BitPos==13]{BatProt_stFltCodAry[AryIdx]=(BatProt_stFltCodAry[AryIdx] | 0x2000);}
  (junction 142) -> (junction 106) [order 1] : [BitPos==11]{BatProt_stFltCodAry[AryIdx]=(BatProt_stFltCodAry[AryIdx] & 0xF7FF);}
  (junction 98) -> (junction 90) [order 2]
  (junction 95) -> (junction 89)
  (junction 142) -> (junction 103) [order 2]
  (junction 106) -> (junction 146)
  (junction 90) -> (junction 89) [order 1] : [BitPos==14]{BatProt_stFltCodAry[AryIdx]=(BatProt_stFltCodAry[AryIdx] | 0x4000);}
  (junction 103) -> (junction 146) [order 1] : [BitPos==12]{BatProt_stFltCodAry[AryIdx]=(BatProt_stFltCodAry[AryIdx] & 0xEFFF);}
  (junction 90) -> (junction 91) [order 2]
  (junction 89) -> (junction 97)
  (junction 103) -> (junction 118) [order 2]
  (junction 146) -> (junction 178)
  (junction 91) -> (junction 97) [order 1] : [BitPos==15]{BatProt_stFltCodAry[AryIdx]=(BatProt_stFltCodAry[AryIdx] | 0x8000);}
  (junction 118) -> (junction 178) [order 1] : [BitPos==13]{BatProt_stFltCodAry[AryIdx]=(BatProt_stFltCodAry[AryIdx] & 0xDFFF);}
  (junction 91) -> (junction 189) [order 2]
  (junction 97) -> (junction 186)
  (junction 118) -> (junction 173) [order 2]
  (junction 178) -> (junction 134)
  (junction 173) -> (junction 134) [order 1] : [BitPos==14]{BatProt_stFltCodAry[AryIdx]=(BatProt_stFltCodAry[AryIdx] & 0xBFFF);}
  (junction 173) -> (junction 174) [order 2]
  (junction 134) -> (junction 156)
  (junction 174) -> (junction 156) [order 1] : [BitPos==15]{BatProt_stFltCodAry[AryIdx]=(BatProt_stFltCodAry[AryIdx] & 0x7FFF);}
  (junction 174) -> (junction 181) [order 2]
  (junction 156) -> (junction 183)
  (junction 181) -> (junction 183)
  (junction 183) -> (junction 189)
  (junction 189) -> (junction 186)
  data: FltFlg input boolean; AryIdx input uint8; BitPos input uint8; BatProt_stFltCodAry data_store_memory size=4

== matlab function ITKLib/Special/ControlAlgorithm/CholCalc ==
  data: In input; Out output
function Out  = CholCalc(In)
%UNTITLED 此处显示有关此函数的摘要
%   此处显示详细说明
Out = chol(In);
end
